simulink model "boat_simulink"  (R2024a)
settings: Solver=FixedStepAuto  StartTime=0.0  StopTime=120  FixedStep=0.01  RelTol=1e-3
settings Model: Creator=gladstonjoseph  LastModifiedBy=gladstonjoseph

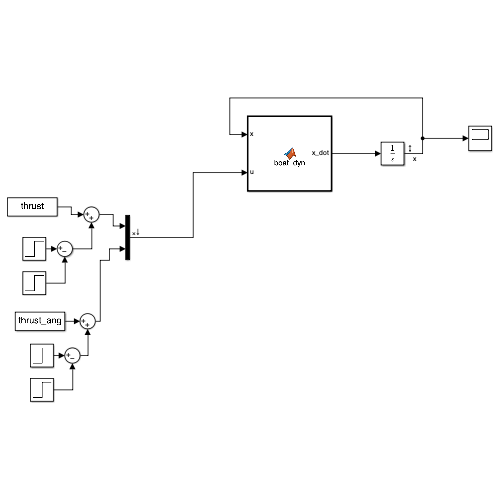
[thumbnail: Simulink's stored preview of the top-level diagram]
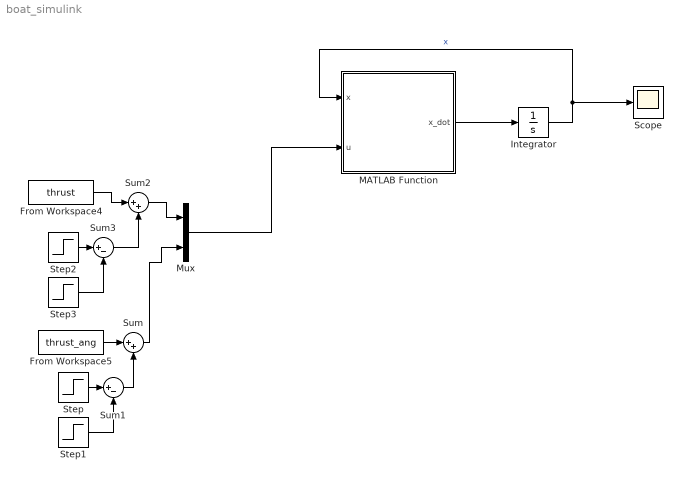
== system boat_simulink ==
  From Workspace4 : FromWorkspace  VariableName=thrust
  From Workspace5 : FromWorkspace  VariableName=thrust_ang
  Integrator : Integrator  InitialCondition=[1, 2, 1.107, 0]'
  MATLAB Function : MATLAB Function  TreatAsAtomicUnit=on
  Mux : Mux  Inputs=2
  Scope : Scope
  Step : Step  Time=5  After=pi/4  SampleTime=0
  Step1 : Step  Time=30  After=pi/4  SampleTime=0
  Step2 : Step  Time=5  After=3  SampleTime=0
  Step3 : Step  Time=30  After=3  SampleTime=0
  Sum : Sum  Inputs=|++
  Sum1 : Sum  Inputs=|+-
  Sum2 : Sum  Inputs=|++
  Sum3 : Sum  Inputs=|+-
  wires:
  Mux/1 -> MATLAB Function/2(u)
  From Workspace4/1 -> Sum2/1
  From Workspace5/1 -> Sum/1
  MATLAB Function/1(x_dot) -> Integrator/1
  Integrator/1 -> Scope/1, MATLAB Function/1(x)  "x"
  Sum/1 -> Mux/2
  Step/1 -> Sum1/1
  Sum1/1 -> Sum/2
  Step1/1 -> Sum1/2
  Sum2/1 -> Mux/1
  Step2/1 -> Sum3/1
  Sum3/1 -> Sum2/2
  Step3/1 -> Sum3/2

== matlab function boat_simulink/MATLAB Function ==
  data: x input; u input; x_dot output
function x_dot = boat_dyn(x, u)
    cd = 0.2;
    cd_rot = 0.4;
    mom_inertia = 1000;
    mass = 300;
    length = 3;

    velocity_x = x(1); velocity_y = x(2); heading = x(3); heading_rate = x(4);
    thrust = u(1); thrust_ang = u(2);

    x_dot = zeros(4, 1);
    x_dot(1) = -(cd/mass) * sqrt(velocity_x^2 + velocity_y^2) * velocity_x + (thrust * cos(thrust_ang+heading));
    x_dot(2) = -(cd/mass) * sqrt(velocity_x^2 + velocity_y^2) * velocity_y + (thrust * sin(thrust_ang+heading));
    x_dot(3) = heading_rate;
    x_dot(4) = -(cd_rot/mom_inertia) * heading_rate^3 - ((thrust*length / mom_inertia) * sin(thrust_ang));


end
